simulink library "UXFD_Lib"  (R2016b)
settings: Solver=ode45  StartTime=0.0  StopTime=10.0  RelTol=1e-3  EnableMultiTasking=on
undefined symbols (not defined in the file): BreakpointData, BreakpointData1, BreakpointData2, BreakpointData_One_A, BreakpointData_Two_A, E2E_P01DataIDMode, E2E_P01ReceiverStatusType, EnumClass, iBit, initalValue, No_Runnable_Period, ObB_EidBsgStDerat_C, p_OVERRIDE_MASTER_SWITCH, SlDemoSign, SwitchOff_P, SwitchOn_P, Table, TableData_M, VCCTi33, VSysD_FidVehDerat1_C
libraries: simulink x28, CCMLib x11, UXFD_Lib x8, canmsglib x2, PTCC_Lib x1, hdlsllib x1
(part 1 of 7)
settings Model: Creator=yaqi.zheng  LastModifiedBy=jichang.liu
settings DataIOCC: LimitDataPoints=on
settings OptimizationCC: LifeSpan=inf
settings DebuggingCC: AllowSymbolicDim=off  SFUnexpectedBacktrackingDiag=warning  SFNoUnconditionalDefaultTransitionDiag=warning  SFExecutionAtInitializationDiag=none
settings GRTTargetCC: TargetLangStandard=C89/C90 (ANSI)  GeneratePreprocessorConditionals=Disable all
settings ConfigComp: CovMetricSettings=dw  CovHtmlReporting=on  CovSaveCumulativeToWorkspaceVar=on  CovSaveSingleToWorkspaceVar=on  CovExternalEMLEnable=off

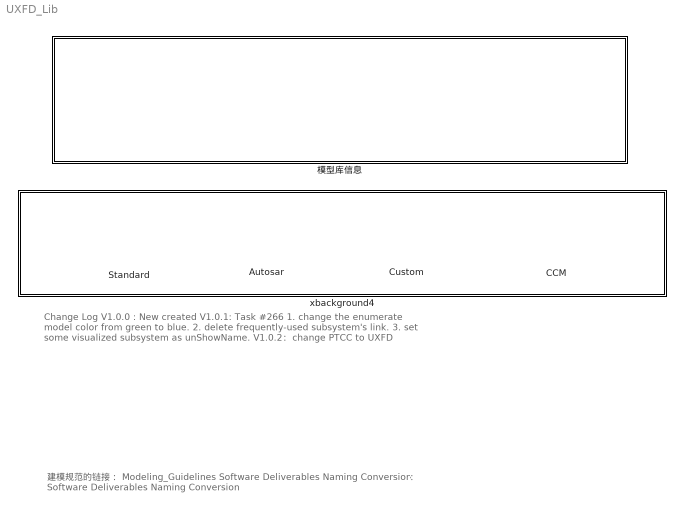
== system UXFD_Lib ==
  note: Change Log
      | V1.0.0 : New created
      |
      | V1.0.1: Task #266
      | 1. change the enumerate model color from green to blue.
      | 2. delete frequently-used subsystem's link.
      | 3. set some visualized subsystem as unShowName.
      | V1.0.2：
      | change PTCC to UXFD
  note: 建模规范的链接：
      | Modeling_Guidelines
      | Software Deliverables Naming Conversion：
      | Software Deliverables Naming Conversion
  Autosar : Subsystem
      mask Display: disp('Autosar')
  CCM : Subsystem
      mask Display: disp('CCM')
  Custom : Subsystem
      mask Display: disp('Custom')
  Standard : Subsystem
      mask Display: disp('Standard')
  xbackground4 : Subsystem
      mask Display: disp(' ')
  模型库信息 : Subsystem  mask(ModelHeader){prj=Geely, desc=UXFD 模型库, ver=1.0.2, date=2019.06.14, rev=0, author=UXFD, matlabver=MATLAB 2016a, simulinkver=MATLAB 2016a, stateflowver=0}
      mask prompts: prj "Project"; desc "Description"; ver "Version"; matlabver "MATLAB Ver"; simulinkver "Simulink Ver"; stateflowver "Stateflow Ver"
      mask init:
      | set_param(gcb, 'LinkStatus', 'none');
      mask Display:
      | plot([0 0 1 1 0],[0.03 1 1 0.03 0.03]) % 内层方框
      | plot([0.5 1],[0.85 0.85]) % 第一条横线
      | plot([0.5 1],[0.7 0.7]) % 第二条横线
      | plot([0.5 1],[0.55 0.55]) % 第三条线横线
      | plot([0.5 1],[0.4 0.4]) % 第四条线横线
      | plot([0 1],[0.25 0.25]) % 第五条横线
      | 
      | plot([0.5 0.5],[0.25 1]) % 第一条竖线
      | plot([0.60 0.60],[0.25 1])% 第二条竖线
      | plot([0.75 0.75],[0.25 1]) % 第三条竖线
      | plot([0.84 0.84],[0.25 1])% 第四条竖线
      | image(imread('geely.png','png'),[0.16 0.33 0.15 0.53]) % 图形位置
      | 
      | text(0.51,0.96,['\fontsize{8}\fontname{Times}\bfProject:'],'verticalAlignment','Top','horizontalAlignment','Left','texmode','on');
      | text(0.62,0.96,['\fontsize{8}\fontname{Times}\rm\fontsize{9}\fontsize{9}' prj],'verticalAlignment','Top','horizontalAlignment','Left','texmode','on');
      | 
      | text(0.51,0.81,['\fontsize{8}\fontname{Times}\bfVersion:' ],'verticalAlignment','Top','horizontalAlignment','Left','texmode','on');
      | text(0.62,0.81,['\fontsize{8}\fontname{Times}' ver],'verticalAlignment','Top','horizontalAlignment','Left','texmode','on');
      | 
      | text(0.51,0.67,['\fontsize{8}\fontname{Times}\bfDate:' ],'verticalAlignment','Top','horizontalAlignment','Left','texmode','on');
      | text(0.62,0.67,['\fontsize{8}\fontname{Times}\rm\fontsize{9}\fontsize{9}' date],'verticalAlignment','Top','horizontalAlignment','Left','texmode','on');
      | 
      | text(0.51,0.51,['\fontsize{8}\fontname{Times}\bfMATLAB Ver:' ],'verticalAlignment','Top','horizontalAlignment','Left','texmode','on');
      | text(0.62,0.51,['\fontsize{8}\fontname{Times}\rm\fontsize{9}\fontsize{9}' matlabver],'verticalAlignment','Top','horizontalAlignment','Left','texmode','on');
      | 
      | text(0.51,0.36,['\fontsize{8}\fontname{Times}\bfStateflow Ver:'],'verticalAlignment','Top','horizontalAlignment','Left','texmode','on');
      | text(0.62,0.36,['\fontsize{8}\fontname{Times}\rm\fontsize{9}\fontsize{9}' stateflowver],'verticalAlignment','Top','horizontalAlignment','Left','texmode','on');
      | %---------------------------------------------------------------------------------
      | text(0.76,0.96,['\fontsize{8}\fontname{Times}\bfAuthor:'],'verticalAlignment','Top','horizontalAlignment','Left','texmode','on');
      | text(0.86,0.96,['\fontsize{8}\fontname{Times}\rm\fontsize{9}\fontsize{9}' author],'verticalAlignment','Top','horizontalAlignment','Left','texmode','on');
      | 
      | text(0.76,0.81,['\fontsize{8}\fontname{Times}\bfRev:'],'verticalAlignment','Top','horizontalAlignment','Left','texmode','on');
      | text(0.86,0.81,['\fontsize{8}\fontname{Times}\rm\fontsize{9}\fontsize{9}' rev],'verticalAlignment','Top','horizontalAlignment','Left','texmode','on');
      | 
      | text(0.76,0.67,['\fontsize{8}\fontname{Times}\bfModel:'],'verticalAlignment','Top','horizontalAlignment','Left','texmode','on');
      | text(0.86,0.67,['\fontsize{8}\fontname{Times}\rm\fontsize{9}\fontsize{9}' desc],'verticalAlignment','Top','horizontalAlignment','Left','texmode','on');
      | 
      | text(0.76,0.51,['\fontsize{8}\fontname{Times}\bfSimulink Ver:'],'verticalAlignment','Top','horizontalAlignment','Left','texmode','on');
      | text(0.86,0.51,['\fontsize{8}\fontname{Times}\rm\fontsize{9}\fontsize{9}' simulinkver],'verticalAlignment','Top','horizontalAlignment','Left','texmode','on');
      | 
      | text(0.01,0.23,['\fontsize{8}\fontname{Times}\bfPROPRIETARY AND CONFIDENTIAL:\rm\fontsize{9}\newline\it\fontsize{10}\fontname{Arial}'                 'Geely Automobile Research Institute. All Right Reserved.'                 ],'verticalAlignment','Top','horizontalAlignment','Left','texmode','on');

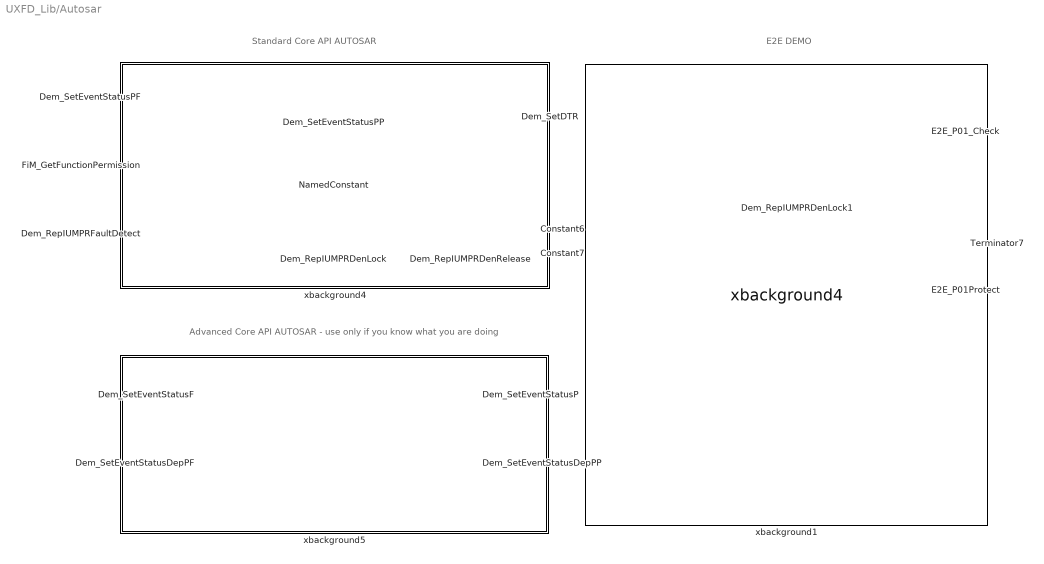
== system UXFD_Lib/Autosar ==
  note: Standard Core API AUTOSAR
  note: Advanced Core API AUTOSAR - use only if you know what you are doing
  note: E2E DEMO
  Constant6 : Constant  Value=72  OutDataTypeStr=Inherit: Inherit via back propagation
      settings: CopyFcn=set_param(gcbh,'ShowName','off');
  Constant7 : Constant  Value=220  OutDataTypeStr=Inherit: Inherit via back propagation
      settings: CopyFcn=set_param(gcbh,'ShowName','off');
  Dem_RepIUMPRDenLock : Subsystem  mask(Dem_RepIUMPRDenLock){}
      mask help: When enabled, this block will block the incrementation the denominator for Ratio Id Vc09XXXX.
      settings: AttributesFormatString=Dem_RepIUMPRDenLock
  Dem_RepIUMPRDenLock1 : PTCC_Lib/Autosar/Dem_RepIUMPRDenLock
      settings: AttributesFormatString=Dem_RepIUMPRDenLock
  Dem_RepIUMPRDenRelease : Subsystem  mask(Dem_RepIUMPRDenRelease){}
      mask help: When enabled, this block will release the incrementation the denominator for Ratio Id Vc09XXXX (i.e. if the conditions are fullfilled for incrementing the denominator for Ratio Id Vc09XXXX, it will be incremented).
      settings: AttributesFormatString=Dem_RepIUMPRDenRelease
  Dem_RepIUMPRFaultDetect : Subsystem  mask(Dem_RepIUMPRFaultDetect){}
      mask help: When enabled, report to the Core BSW, that Ratio Id Vc09XXXX has been able to detect a fault (increment Numerator for Ratio Id Vc09XXXX)
      settings: AttributesFormatString=Dem_RepIUMPRFaultDetect
  Dem_SetDTR : Subsystem  Description="API method to update mode $06 testdata.                                       Dem_SetDTR(UInt16 DTRId, sint32 TestVal, sint32 LowerLimit, sint32  UpperLimit, Ctrlval )"  mask(Vcc_SetDTR){lsb=1.0, offset=0}
      mask help:
      | Reports a DTR result with lower and upper limit.
      | The types of the TestValue and it limits should be Float32.
      | The test value and test limits are converted to Int32s using the
      | lsb and offset parameters in this block
      |
      | API is needed in OBD-relevant ECUs only
      settings: AttributesFormatString=Vcc_SetDTR
  Dem_SetEventStatusDepPF : Subsystem  TreatAsAtomicUnit=on  mask(Dem_SetEventStatusDepPre-Failed){}
      mask help:
      | Only to be used by dependability functions.
      | When enabled, events with status Pre-Failed is sent to the Diagnostic Core
      settings: AttributesFormatString=Dem_SetEventStatusDep\nPre-Failed
  Dem_SetEventStatusDepPP : Subsystem  TreatAsAtomicUnit=on  mask(Dem_SetEventStatusDepPre-Passed){}
      mask help:
      | Only to be used by dependability functions.
      | When enabled, events with status Pre-Passed is sent to the Diagnostic Core
      settings: AttributesFormatString=Dem_SetEventStatusDep\nPre-Passed
  Dem_SetEventStatusF : Subsystem  TreatAsAtomicUnit=on  mask(Dem_SetEventStatusFailed){}
      mask help: When enabled, events with status Failed is sent to the Diagnostic Core
      settings: AttributesFormatString=Dem_SetEventStatus\nFailed
  Dem_SetEventStatusP : Subsystem  mask(Dem_SetEventStatusPassed){}
      mask help: When enabled, events with status Passed is sent to the Diagnostic Core
      settings: AttributesFormatString=Dem_SetEventStatus\nPassed
  Dem_SetEventStatusPF : Subsystem  mask(Dem_SetEventStatusPre-Failed){}
      mask help: When enabled, events with status Pre-Failed is sent to the Diagnostic Core
      settings: AttributesFormatString=Dem_SetEventStatus\nPre-Failed
  Dem_SetEventStatusPP : Subsystem  mask(Dem_SetEventStatusPre-Passed){}
      mask help: When enabled, events with status Pre-Passed is sent to the Diagnostic Core
      settings: AttributesFormatString=Dem_SetEventStatus\nPre-Passed
  E2E_P01Protect : Subsystem
  E2E_P01_Check : Subsystem
  FiM_GetFunctionPermission : Subsystem  mask(FiM_GetFunctionPermission){}
      mask help:
      | When enabled, this block ask the core for permission to execute a monitor with the FID.
      | Note: If this is used for activating reconfigurations, Perm == 0 => Activate reconfiguration.
      settings: AttributesFormatString=FiM_GetFunctionPermission
  NamedConstant : Subsystem  mask(NamedConstant){const_name=VcEvName}
      mask prompts: const_name "Constant Name"
      mask help:
      | Enter a name for a preprocessor defined constant.
      | The following naming convention shall be used:
      | These prefixes shall be used for the following IDs (without underscores):
      | VcEv - Event IDs
      | VcFi - Function IDs (FiD)
      | VcRv - Ranking Value IDs
      | Vc06 - Mode $06 Test result IDs
      | Vc09 - IU(M)PR IDs (Mode $09)
      |
      | E.g.
      | VcEvBoostHigh - An event ID name for too high boost pressure
      | VcFiBoostPeak - A FiD for the Peak pressure boost monitor
      settings: AttributesFormatString=Named Constant
      mask Display: text(0.5, 0.5, get_param(gcb, 'const_name'), 'horizontalAlignment', 'center')
  Terminator7 : Terminator
  xbackground1 : UXFD_Lib/Autosar/xbackground4  SystemSampleTime=-1
  xbackground4 : Subsystem
      mask Display: disp(' ')
  xbackground5 : Subsystem
      mask Display: disp(' ')
  wires:
  E2E_P01Protect/1(E2E_P01Protect_ReturnType) -> Terminator7/1
  Constant6/1 -> E2E_P01Protect/1(DataLength)
  Constant7/1 -> E2E_P01Protect/2(DataID)

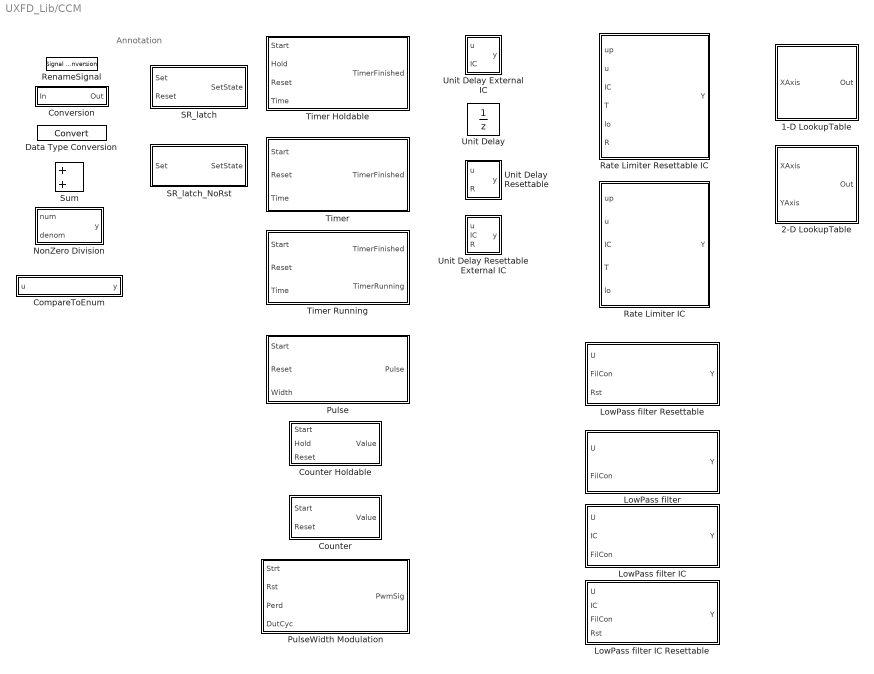
== system UXFD_Lib/CCM ==
  note: Annotation
  1-D LookupTable : Subsystem  mask(1D Lookup table NGCC v1.1){TableData=[4 7 6], TableDataDataType=Inherit: auto, BreakpointsXAxis=[1:3], BreakpointsXAxisDataType=Inherit: auto}
      mask help:
      | NGCC version of the Simulink standard 2-D lookup table.
      | "X-axis" is used as notation instead of "breakpoints 1".
      | Deviation from standard 2-D lookup table default settings:
      | - Extrapolation method: Clip, use last table value for inputs at or above last breakpoint.
      | - Saturate on integer overflow.
      | - Integer rounding mode: Floor
      | - Does NOT require all inputs to have the same data type
      |
      | Mx-VDev tested: Yes
      mask init:
      | blkNameMask = gcb;
      | 
      | % Redraw block at resize
      | set_param(blkNameMask,'MaskRunInitForIconRedraw','on')
      mask Display:
      | pos = get_param(gcb, 'Position');
      | width = pos(3) - pos(1);
      | height = pos(4) - pos(2);
      | doPlot = true;
      | blockHandle = gcb;
      | try
      |     tableDialogText = get_param(blockHandle,'TableData');
      |     try
      |         table = evalin('base',tableDialogText);
      |         tableValue = table.Value;
      |     catch
      |         tableValue = recursiveMaskParameterSearch(blockHandle,tableDialogText);
      |     end
      |     breakpointsXAxisDialogText = get_param(blockHandle,'BreakpointsXAxis');
      |     try
      |         breakpointsXAxisHandle = evalin('base',breakpointsXAxisDialogText);
      |         bp1 = breakpointsXAxisHandle.Value;
      |     catch
      |         bp1 = recursiveMaskParameterSearch(blockHandle,breakpointsXAxisDialogText);
      |     end
      | catch
      |     tableValue = str2num(get_param(blockHandle,'TableData'));
      |     bp1 = str2num(get_param(blockHandle,'BreakpointsXAxis'));
      |     doPlot = true;
      |     if (isempty(tableValue) || isempty(bp1))
      |         doPlot = false;
      |     end
      | end
      | if doPlot
      |     % Scale table and breakpoint data to fit block icon size
      |     if min(tableValue(:)) == max(tableValue(:))
      |         tableScaleTemp2 = ones(size(tableValue))*10;
      |     else
      |         tableScaleTemp1 = tableValue-min(tableValue(:));
      |         tableScaleTemp2 = (tableScaleTemp1/(max(tableScaleTemp1(:))-min(tableScaleTemp1(:))))*((height-5)-10);
      |     end
      |     tableScaled = tableScaleTemp2 + 5;
      | 
      |     if min(bp1(:)) == max(bp1(:))
      |         bp1ScaleTemp2 = bp1;
      |     else
      |         bp1ScaleTemp1 = bp1-min(bp1(:));
      |         bp1ScaleTemp2 = (bp1ScaleTemp1/(max(bp1ScaleTemp1(:))-min(bp1ScaleTemp1(:))))*((width-5)-12);
      |     end
      |     bp1Scaled = bp1ScaleTemp2 + 12;
      | 
      |     % plot data
      |     for i=1:length(tableValue(:,1))
      |         try
      |             plot(bp1Scaled,tableScaled(i,:))
      |         catch
      |             disp(num2str(tableScaled(i,:)))
      |         end
      |     end
      | 
      | else
      |     disp('Input data\nError')
      | end
      | % plot axis
      | plot([12 12],[5 height-10])
      | plot([12 width-5],[5 5])
      | 
      | port_label('input',1,'X')
      | text(width/2-20,height-7,'1-D T(x)')
  2-D LookupTable : Subsystem  mask(2D Lookup table NGCC v1.1){TableData=[4 5 6;16 19 20;10 18 23], TableDataDataType=Inherit: auto, BreakpointsXAxis=[1:3], BreakpointsXAxisDataType=Inherit: auto, BreakpointsYAxis=[1:3], BreakpointsYAxisDataType=Inherit: auto}
      mask help:
      | NGCC version of the Simulink standard 2-D lookup table.
      | "X- and Y-axis" is used as notation instead of "breakpoints 1" and "breakpoints 2".
      | Deviation from standard 2-D lookup table default settings:
      | - Extrapolation method: Clip, use last table value for inputs at or above last breakpoint.
      | - Saturate on integer overflow.
      | - Integer rounding mode: Floor
      | - Does NOT require all inputs to have the same data type
      |
      | Mx-VDev tested: Yes
      mask init:
      | blkNameMask = gcb;
      | 
      | % Redraw block at resize
      | set_param(blkNameMask,'MaskRunInitForIconRedraw','on')
      mask Display:
      | pos = get_param(gcb, 'Position');
      | width = pos(3) - pos(1);
      | height = pos(4) - pos(2);
      | doPlot = true;
      | blockHandle = gcb;
      | try
      |     tableDialogText = get_param(blockHandle,'TableData');
      |     try
      |         table = evalin('base',tableDialogText);
      |         tableValue = table.Value;
      |     catch
      |         tableValue = recursiveMaskParameterSearch(blockHandle,tableDialogText);
      |     end
      |     breakpointsYAxisDialogText = get_param(blockHandle,'BreakpointsYAxis');
      |     try
      |         breakpointsYAxisHandle = evalin('base',breakpointsYAxisDialogText);
      |         bp2 = breakpointsYAxisHandle.Value;
      |     catch
      |         bp2 = recursiveMaskParameterSearch(blockHandle,breakpointsYAxisDialogText);
      |     end
      |     breakpointsXAxisDialogText = get_param(blockHandle,'BreakpointsXAxis');
      |     try
      |         breakpointsXAxisHandle = evalin('base',breakpointsXAxisDialogText);
      |         bp1 = breakpointsXAxisHandle.Value;
      |     catch
      |         bp1 = recursiveMaskParameterSearch(blockHandle,breakpointsXAxisDialogText);
      |     end
      | catch
      |     tableValue = str2num(get_param(blockHandle,'TableData'));
      |     bp2 = str2num(get_param(blockHandle,'BreakpointsYAxis'));
      |     bp1 = str2num(get_param(blockHandle,'BreakpointsXAxis'));
      |     doPlot = true;
      |     if (isempty(tableValue) || isempty(bp1) || isempty(bp2))
      |         doPlot = false;
      |     end
      | end
      | if doPlot
      |     % Scale table and breakpoint data to fit block icon size
      |     if min(tableValue(:)) == max(tableValue(:))
      |         tableScaleTemp2 = ones(size(tableValue))*10;
      |     else
      |         tableScaleTemp1 = tableValue-min(tableValue(:));
      |         tableScaleTemp2 = (tableScaleTemp1/(max(tableScaleTemp1(:))-min(tableScaleTemp1(:))))*((height-5)-10);
      |     end
      |     tableScaled = tableScaleTemp2 + 5;
      | 
      |     if min(bp1(:)) == max(bp1(:))
      |         bp1ScaleTemp2 = bp1;
      |     else
      |         bp1ScaleTemp1 = bp1-min(bp1(:));
      |         bp1ScaleTemp2 = (bp1ScaleTemp1/(max(bp1ScaleTemp1(:))-min(bp1ScaleTemp1(:))))*((width-5)-12);
      |     end
      |     bp1Scaled = bp1ScaleTemp2 + 12;
      | 
      |     % plot data
      |     for i=1:length(tableValue(:,1))
      |         try
      |             plot(bp1Scaled,tableScaled(i,:))
      |         catch
      |             disp(num2str(tableScaled(i,:)))
      |         end
      |     end
      | 
      | else
      |     disp('Input data\nError')
      | end
      | % plot axis
      | plot([12 12],[5 height-10])
      | plot([12 width-5],[5 5])
      | 
      | port_label('input',1,'X')
      | port_label('input',2,'Y')
      | text(width/2-20,height-7,'2-D T(x,y)')
  CompareToEnum : Subsystem  mask(Compare to Enum NGCC v1.0){relop===, const=EnumClass.Value, OutDataTypeStr=boolean, ZeroCross=on}
      mask prompts: relop "Simulink:masks:Operator_MP"; const "Simulink:masks:ConstantValue_MP"; OutDataTypeStr "Simulink:masks:OutputDataType_MP"; ZeroCross "Simulink:masks:EnableZerocrossingDetection_MP"
      mask help:
      | Compare to an Enum. Enum class is hidden from the mask i.e. displays only the value if the Enum is defined.
      |
      | Mx-VDev tested: Yes
      mask init:
      | blkName = gcb;
      | 
      | if strcmp(get_param(gcbh,'OutDataTypeStr'),'boolean')
      | 	setValue = 'boolean';
      | else
      | 	setValue = 'fixdt(0, 8)';
      | end
      | 
      | set_param([blkName,'/Compare'],'relop',relop, ...
      | 	'OutDataTypeStr', setValue, 'ZeroCross', ZeroCross);
      | 
      | str = [relop,' C']; %default
      | 
      | const_str = get_param(blkName, 'const');
      | 
      | if isempty(strfind(const_str, ' ')) && isempty(strfind(const_str, ','))
      |     % scalar or single expression
      |     if isempty(str2num(const_str))
      |         %expression
      |         str = [relop, ' ', const_str];
      |     elseif length(const) == 1
      |         if ismethod(const,'addClassNameToEnumNames') % Enum
      |             str = [relop,' ',char(const)];
      |         else
      |             str = [relop,' ',num2str(double(const))];
      |         end
      |     end
      | end
      mask TypeOptions relop: == | ~= | < | <= | >= | >
      mask TypeOptions OutDataTypeStr: uint8 | boolean
      mask Callback ZeroCross: sl('zeroCrossEnable', gcbh);
      mask Display: disp(str)
  Conversion : Subsystem  mask(Data Type Conversion NGCC v1.1){outputDataType=Inherit: Inherit via back propagation}
      mask prompts: outputDataType "Convert data type to:"
      mask help:
      | CCM version of the standard Simulink block.
      | This version displays the output data type name on the block icon, regardless of data type.
      |
      | Mx-VDev tested: Yes
      mask Display:
      | if strcmp(char(get_param(gcb,'MaskValues')),'Inherit: Inherit via back propagation')
      |     disp('Conversion')
      | else
      |     disp(char(get_param(gcb,'MaskValues')))
      | end
  Counter : Subsystem  mask(Counter NGCC v1.0){}
      mask help:
      | If Start (1) is true, the counter is started.
      | Counter will be reset to 0 and stopped if Reset (2) is true.
      | This block is reset dominant.
      | Value (output) specifies the counter value, data type VCCUInt32.
      |
      | Mx-VDev tested: Yes
      mask Display:
      | try
      |     image(imread([CCMConfig.GetRootDir '\Shared\SimulinkLibrary\Images\counter.bmp']))
      | catch
      |     fprintf('Counter\nHoldable')
      | end
      | port_label('output',1,'Value')
      | port_label('input',1,'Start')
      | port_label('input',2,'Reset')
  Counter Holdable : Subsystem  mask(Counter Holdable NGCC v1.0){}
      mask help:
      | If Start (1) is true, the counter is started.
      | Counter will continue counting until Hold (2) is true, then the counter value will be held.
      | Counter will be reset to 0 if Reset (3) is true.
      | Value (output) specifies the counter value, data type VCCUInt32.
      |
      | Mx-VDev tested: Yes
      mask Display:
      | try
      |     image(imread([CCMConfig.GetRootDir '\Shared\SimulinkLibrary\Images\counter.bmp']))
      | catch
      |     fprintf('Counter\nHoldable')
      | end
      | port_label('output',1,'Value')
      | port_label('input',1,'Start')
      | port_label('input',2,'Hold')
      | port_label('input',3,'Reset')
  Data Type Conversion : DataTypeConversion  SaturateOnIntegerOverflow=on
      settings: AttributesFormatString=%<OutDataTypeStr>
  LowPass filter : Subsystem  mask(Low-pass filter NGCC v1.0){InputOutputDataType=single, FilterConstantDataType=VCCTi33, RunnablePeriod=No_Runnable_Period}
      mask prompts: InputOutputDataType "Input/Output Data Type"; FilterConstantDataType "Filter Time Constant Data Type:"; RunnablePeriod "SWC Sampling Time Parameter:"
      mask help:
      | Typical NGCC low-pass filter with filter length 1.
      | U is the input signal that is to be filtered.
      | FilCon is the filter time constant.
      | Y is the filtered output.
      |
      | Mx-VDev tested: Yes
      mask init:
      | blkNameMask = gcb;
      | IODataType = get_param(blkNameMask,'InputOutputDataType');
      | if strcmp(IODataType,'single')
      |     dataTypeSlope = 2^(-12);
      | else
      |     try
      |     dataTypeSlope = evalin('base',[IODataType '.Slope']); %Fixed point
      |     catch
      |         dataTypeSlope = 1; %Integer
      |     end
      | end
      | %Set sampletime
      | blkName = gcb;
      | modelName = char(regexp(blkName,'(\w*)_(?:Runnable|lib)','tokens','once'));
      | if isempty(modelName)
      |     modelName = 'No';
      | end
      | timeParameter = [modelName '_Runnable_Period'];
      | set_param(blkName, 'RunnablePeriod',timeParameter);
      mask Display: disp(['Y = U[n]*k + Y[n-1]*(1-k)' char(uint16(10)) 'n: sample' char(uint16(10)) 'k: filter constant' char(uint16(10)) 'Init value = U[0]']);
  LowPass filter Resettable : Subsystem  mask(Low-pass filter Resettable NGCC v1.0){InputOutputDataType=single, FilterConstantDataType=VCCTi33, RunnablePeriod=No_Runnable_Period}
      mask prompts: InputOutputDataType "Input/Output Data Type"; FilterConstantDataType "Filter Time Constant Data Type:"; RunnablePeriod "SWC Sampling Time Parameter:"
      mask help:
      | Typical NGCC low-pass filter with filter length 1.
      | U is the input signal that is to be filtered.
      | FilCon is the filter time constant.
      | Rst is the filter reset condition (boolean).
      | Y is the filtered output.
      |
      | Mx-VDev tested: Yes
      mask init:
      | %Set sample time
      | blkName = gcb;
      | modelName = char(regexp(blkName,'(\w*)_(?:Runnable|lib)','tokens','once'));
      | if isempty(modelName)
      |     modelName = 'No';
      | end
      | timeParameter = [modelName '_Runnable_Period'];
      | set_param(blkName, 'RunnablePeriod',timeParameter);
      mask Display: disp(['Y = U[n]*k + Y[n-1]*(1-k)' char(uint16(10)) 'n: sample' char(uint16(10)) 'k: filter constant' char(uint16(10)) 'Init value = U[0]']);
  LowPass filter IC : Subsystem  mask(Low-pass filter IC NGCC v1.0){InputOutputDataType=single, FilterConstantDataType=VCCTi33, RunnablePeriod=No_Runnable_Period}
      mask prompts: InputOutputDataType "Input/Output Data Type"; FilterConstantDataType "Filter Time Constant Data Type:"; RunnablePeriod "SWC Sampling Time Parameter:"
      mask help:
      | Typical NGCC low-pass filter with filter length 1.
      | U is the input signal that is to be filtered.
      | IC is the initial condition value.
      | FilCon is the filter time constant.
      | Y is the filtered output.
      |
      | Mx-VDev tested: No
      mask init:
      | blkNameMask = gcb;
      | IODataType = get_param(blkNameMask,'InputOutputDataType');
      | if strcmp(IODataType,'single')
      |     dataTypeSlope = 2^(-12);
      | else
      |     try
      |     dataTypeSlope = evalin('base',[IODataType '.Slope']); %Fixed point
      |     catch
      |         dataTypeSlope = 1; %Integer
      |     end
      | end
      | 
      | %Set sample time
      | blkName = gcb;
      | modelName = char(regexp(blkName,'(\w*)_(?:Runnable|lib)','tokens','once'));
      | if isempty(modelName)
      |     modelName = 'No';
      | end
      | timeParameter = [modelName '_Runnable_Period'];
      | set_param(blkName, 'RunnablePeriod',timeParameter);
      mask Display: disp(['Y = U[n]*k + Y[n-1]*(1-k)' char(uint16(10)) 'n: sample' char(uint16(10)) 'k: filter constant' char(uint16(10)) 'Init value = IC']);
  LowPass filter IC Resettable : Subsystem  mask(Low-pass filter IC Resettable NGCC v1.0){InputOutputDataType=single, FilterConstantDataType=VCCTi33, RunnablePeriod=No_Runnable_Period}
      mask prompts: InputOutputDataType "Input/Output Data Type"; FilterConstantDataType "Filter Time Constant Data Type:"; RunnablePeriod "SWC Sampling Time Parameter:"
      mask help:
      | Typical NGCC low-pass filter with filter length 1.
      | IC is the initial condition (value).
      | U is the input signal that is to be filtered.
      | FilCon is the filter time constant.
      | Rst is the filter reset condition (boolean).
      | Y is the filtered output.
      |
      | Mx-VDev tested: No
      mask init: same as UXFD_Lib/CCM/LowPass filter Resettable
      mask Display: disp(['Y = U[n]*k + Y[n-1]*(1-k)' char(uint16(10)) 'n: sample' char(uint16(10)) 'k: filter constant' char(uint16(10)) 'Init value = IC']);
  NonZero Division : Subsystem  mask(Non Zero Division NGCC v1.3){dataTypeNum=single, dataTypeDen=single, dataTypeOut=single}
      mask prompts: dataTypeNum "Data type of numerator"; dataTypeDen "Data type of denominator"; dataTypeOut "Data type of output"
      mask help:
      | Performs a division that is protected against division by zero.
      | First input is numerator, second input is denominator.
      | User must enter the data types of the two input signals as well as the output signal.
      |
      | Mx-VDev tested: Yes
      mask init:
      | blkNameMask = gcb;
      | DenominatorDataType = get_param(blkNameMask,'dataTypeDen');
      | if strcmp(DenominatorDataType,'single')
      |     dataTypeSlope = 2^(-100);
      | else
      |     try
      |         dataTypeSlope = evalin('base',[DenominatorDataType '.Slope']); %Fixed point
      |     catch
      |         dataTypeSlope = 1; %Integer
      |     end
      | end
      mask Display:
      | port_label('output',1,'y')
      | port_label('input',1,'x')
      | port_label('input',2,'÷')
      | fprintf('Non-Zero\nDivision')
  Pulse : Subsystem  mask(Pulse NGCC v1.0){timeDataType=VCCTi33, RunnablePeriod=No_Runnable_Period}
      mask prompts: timeDataType "Pulse width data type (s):"; RunnablePeriod "SWC Sampling Time Parameter:"
      mask help:
      | If Start (1) is true, the Pulse (output) is started.
      | If Start is set during [Pulse == true], the timer is reset and the Pulse is kept true.
      | Pulse will be reset to 0 if Reset (2) is true.
      | Width (3) defines the pulse width in seconds.
      | If Width is set to zero, Pulse will be set to false.
      | Reset is always master over Start.
      |
      | Mx-VDev tested: Yes
      mask init: same as UXFD_Lib/CCM/LowPass filter Resettable
      mask Display:
      | x=[0.2 0.35 0.35 0.65 0.65 0.8];
      | y=[0.2 0.2 0.7 0.7 0.2 0.2];
      | plot(x,y)
  PulseWidth Modulation : Subsystem  mask(PulseWidth Modulation NGCC v1.0){timeDataType=VCCTi33, RunnablePeriod=No_Runnable_Period}
      mask prompts: timeDataType "Period time input data type:"; RunnablePeriod "SWC Sampling Time Parameter:"
      mask help:
      | If Start(1) is true the pulse generator is started.
      | It will continue to run until Reset(2) is true. It will start again when Reset is set to false.
      | Data type of Period time(3) and the SWC Sampling Time has to be specified in the mask.
      | Data type of Duty Cycle(4) is VCCPerc30 and determines the ratio of the period time when the signal is true.
      | The period starts with the duty cycle, i.e. the signal is first true after reset or start.
      | Default value, when pulse generator is not started or when it is held with the reset function, is true.
      |
      | Mx-VDev tested: Yes
      mask init: same as UXFD_Lib/CCM/LowPass filter Resettable
      mask Display:
      | x=[0.1 1 1 2.1 2.1 3 3 4.1 4.1 5 5 6.1 6.1 7 7 8.1] * 10 + 30;
      | y=[1 1 0 0 1 1 0 0 1 1 0 0 1 1 0 0] * 15 + 30;
      | plot(x,y)
  Rate Limiter IC : Subsystem  mask(Rate Limiter Dynamic IC NGCC v1.0){InputOutputDataType=single}
      mask prompts: InputOutputDataType "Data type inputs/output:"
      mask help:
      | Limit rising and falling rates of the input signal.
      | up: upper rate limit
      | u: input signal to be rate limited
      | IC: initial condition
      | T: SWC runnable period
      | lo: lower rate limit (input should be negative)
      |
      | The rates 'up' and 'lo' should be per second (*/s), since the block converts seconds to sample before calculations.
      |
      | Mx-VDev tested: Yes
      mask Display: plot([0.15 0.95],[.5 .5],[.5 .5],[0.05 0.95],0.05+0.9*[.2 .8],0.05+0.9*[0 1]);
  Rate Limiter Resettable IC : Subsystem  mask(Rate Limiter Dynamic Resettable IC NGCC v1.0){InputOutputDataType=single}
      mask prompts: InputOutputDataType "Data type inputs/output:"
      mask help:
      | Limit rising and falling rates of the input signal.
      | up: upper rate limit
      | u: input signal to be rate limited
      | IC: initial condition
      | T: SWC runnable period
      | lo: lower rate limit
      | R: reset flag, resets to the initial condition
      |
      | The rates 'up' and 'lo' should be per second (*/s), since the block converts seconds to sample before calculations.
      |
      | Mx-VDev tested: Yes
      mask Display: plot([0.15 0.95],[.5 .5],[.5 .5],[0.05 0.95],0.05+0.9*[.2 .8],0.05+0.9*[0 1]);
  RenameSignal : SignalConversion  OverrideOpt=on  mask(Rename signal NGCC v1.1){}
      mask help:
      | Typically used when bus signals are relayed.
      |
      | Mx-VDev tested: Yes
      mask Display: fprintf('Rename')
  SR_latch : Subsystem  mask(SR-latch NGCC v1.0){}
      mask help:
      | Set/reset-latch with default value 0 (false).
      | S   R   Q
      | ----------
      | 0   0   Q[n-1]
      | 0   1   0
      | 1   0   1
      | 1   1   0
      |
      | where Q[n-1] is the previous output value.
      |
      | Mx-VDev tested: Yes
  SR_latch_NoRst : Subsystem  mask(SR-latch-no-reset NGCC v1.0){}
      mask help:
      | Set-latch with default value 0 (false).
      | S   Q
      | ----------
      | 0   Q[n-1]
      | 1   1
      |
      | where Q[n-1] is the previous output value.
      |
      | Mx-VDev tested: Yes
  Sum : Sum  SaturateOnIntegerOverflow=on  InputSameDT=on
  Timer : Subsystem  mask(Timer NGCC v1.0){timeDataType=VCCTi33, RunnablePeriod=No_Runnable_Period}
      mask prompts: timeDataType "Time data type:"; RunnablePeriod "SWC Sampling Time Parameter:"
      mask help:
      | If Start (1) is true, the timer is started.
      | The timer works as a "set/reset"-functionality, i.e. start does not have to be "true" continuously to keep the timer running.
      | Timer will be reset to 0 if Reset (2) is true.
      | TimerFinished (output) specifies if the timer is finished (boolean).
      | If Time (3) is set to zero, this block will function as a set-reset latch.
      | Reset is always master over Start.
      |
      | Mx-VDev tested: Yes
      mask init: same as UXFD_Lib/CCM/LowPass filter Resettable
      mask Display:
      | try
      |     image(imread([CCMConfig.GetRootDir '\Shared\SimulinkLibrary\Images\timer.bmp']))
      | catch
      |     fprintf('Timer\nHoldable')
      | end
      | port_label('output',1,'TmrFinshd')
      | port_label('input',1,'Start')
      | port_label('input',2,'Reset')
      | port_label('input',3,'Time')
  Timer Holdable : Subsystem  mask(Timer Holdable NGCC v1.1){timeDataType=VCCTi33, RunnablePeriod=No_Runnable_Period}
      mask prompts: timeDataType "Time data type:"; RunnablePeriod "SWC Sampling Time Parameter:"
      mask help:
      | If Start (1) is true, the timer is started.
      | Timer will continue running until Hold (2) is true, then the timer value will be held.
      | If Hold becomes false, the timer will continue when conditions to start is fulfilled.
      | The Start and Hold serve as a "set/reset"-functionality, i.e. start does not have to be "true" continuously to keep the timer running.
      | Timer will be reset to 0 if Reset (3) is true.
      | TimerFinished (output) specifies if the timer is finished (boolean).
      | If Time is set to zero, this block will function as a set-reset latch.
      | Hold and Reset are always master over Start.
      |
      | Mx-VDev tested: Yes
      mask init: same as UXFD_Lib/CCM/LowPass filter Resettable
      mask Display:
      | try
      |     image(imread([CCMConfig.GetRootDir '\Shared\SimulinkLibrary\Images\timer.bmp']))
      | catch
      |     fprintf('Timer\nHoldable')
      | end
      | port_label('output',1,'TmrFinshd')
      | port_label('input',1,'Start')
      | port_label('input',2,'Hold')
      | port_label('input',3,'Reset')
      | port_label('input',4,'Time')
  Timer Running : Subsystem  mask(Timer Running NGCC v1.0){timeDataType=VCCTi33, RunnablePeriod=No_Runnable_Period}
      mask prompts: timeDataType "Time data type:"; RunnablePeriod "SWC Sampling Time Parameter:"
      mask help:
      | If Start (1) is true, the timer is started.
      | The timer works as a "set/reset"-functionality, i.e. start does not have to be "true" continuously to keep the timer running.
      | Timer will be reset to 0 if Reset (2) is true.
      | TimerFinished (output) specifies if the timer is finished (boolean).
      | If Time (3) is set to zero, this block will function as a set-reset latch.
      | Reset is always master over Start.
      |
      | TmrRunng (output 2) will be set when timer is activated.
      |
      | Mx-VDev tested: Yes
      mask init: same as UXFD_Lib/CCM/LowPass filter Resettable
      mask Display:
      | try
      |     image(imread([CCMConfig.GetRootDir '\Shared\SimulinkLibrary\Images\timer.bmp']))
      | catch
      |     fprintf('Timer\nHoldable')
      | end
      | port_label('output',1,'TmrFinshd')
      | port_label('output',2,'TmrRunng')
      | port_label('input',1,'Start')
      | port_label('input',2,'Reset')
      | port_label('input',3,'Time')
  Unit Delay : UnitDelay  InitialCondition=initalValue  SampleTime=-1
      settings: AttributesFormatString=X0=%<X0>
  Unit Delay External IC : Subsystem  mask(Unit Delay External Initial Condition NGCC v1.0){dataType=single}
      mask prompts: dataType "Data type:"
      mask help:
      | NGCC version of the Simulink built-in block with data type control and boolean datatype usage for internal switch condition.
      | -----------------------------------------------------
      | Normally, the output is the signal u delayed by one sample period.
      | The initial condition is given by the signal IC.
      |
      | Mx-VDev tested: Yes
      mask Display: dpoly(1,[1 0],'z')
  Unit Delay Resettable : Subsystem  mask(Unit Delay Resettable NGCC v1.0){initialCondition=0, dataType=single}
      mask prompts: initialCondition "Initial condition:"; dataType "Data type:"
      mask help:
      | NGCC version of the Simulink built-in block with data type control and boolean datatype usage for internal switch condition.
      | -----------------------------------------------------
      | Normally, the output is the signal u delayed by one sample period.
      | When the reset signal R is true, the state and the output are always set equal to the initial condition parameter.  This reset action is vectorized and supports scalar expansion.
      |
      | Mx-VDev tested: Yes
      settings: AttributesFormatString=X0=%<initialCondition>
      mask Display: dpoly(1,[1 0],'z')
  Unit Delay Resettable External IC : Subsystem  mask(Unit Delay Resettable External Initial Condition NGCC v1.0){dataType=single}
      mask prompts: dataType "Data type:"
      mask help:
      | NGCC version of the Simulink built-in block with data type control and boolean datatype usage for internal switch condition.
      | -----------------------------------------------------
      | Normally, the output is the signal u delayed by one sample period.
      | When the reset signal R is true, the state and the output are always set equal to the initial condition signal IC.  This reset action is vectorized and supports scalar expansion.
      |
      | Mx-VDev tested: Yes
      mask Display: dpoly(1,[1 0],'z')

== system UXFD_Lib/Custom ==
  CAN : Subsystem
      mask Display: disp('CAN')
  Diagnose : Subsystem
      mask Display: disp('Diagnose')
  PIN : Subsystem
      mask Display: disp('PIN')
  xbackground4 : UXFD_Lib/xbackground4  SystemSampleTime=-1

== system UXFD_Lib/Standard ==
  Bit Operation : Subsystem
      settings: CopyFcn=set_param(gcbh,'ShowName','off');
      mask Display: disp('Bit Operation')
  Calibration : Subsystem
      settings: CopyFcn=set_param(gcbh,'ShowName','off');
      mask Display: disp('Calibration')
  Discrete dynamics : Subsystem
      settings: CopyFcn=set_param(gcbh,'ShowName','off');
      mask Display: disp('Discrete dynamics')
  Math : Subsystem
      mask Display: disp('Math')
  Relation&Logic : Subsystem
      mask Display: disp('Relation & Logic')
  Signals and systems : Subsystem
      mask Display: disp('Signals and systems')
  xbackground4 : UXFD_Lib/xbackground4  SystemSampleTime=-1

== system UXFD_Lib/xbackground4 ==

== system UXFD_Lib/模型库信息 ==

== system UXFD_Lib/Autosar/Dem_RepIUMPRDenLock ==
  Vc09 : Inport
  EntryCond : EnablePort
  Dem_RepIUMPRDenLock : S-Function  FunctionName=Dem_RepIUMPRDenLock_flp  Parameters=dt  SFunctionDeploymentMode=off  EnableBusSupport=off  mask(TL_CustomCode){data={'#state',0,'#param',0,'#work',0,'codefile','Dem_RepIUMPRDenLock.c','prodcode',0,'logdata',{'plotchannels',[]},'output',{'name','$S_ok','varname','ok','type','Bool'},'input',{'name','$S_RatioId','varname','RatioId','type','UInt16'},'date',735300.29244876152}, dt=-1}
      mask help:
      | TargetLink Custom Code block:
      | Allows to insert custom code into a TargetLink application.
      settings: AttributesFormatString=Dem_RepIUMPRDenLock  DeleteFcn=if exist('delete_tlblock','file')==2,delete_tlblock(gcbh);end  NameChangeFcn=if exist('rename_tlblock','file')==2,rename_tlblock(gcbh);end  OpenFcn=if exist('tl_open_blockdlg','file')==2,tl_open_blockdlg(gcbh);else,open_system(gcbh,'mask');end
      mask Help: eval(['tl_online_help(''Topic'',''',get_param(gcbh,'MaskType'),''')'])
      mask Display:
      | plot([-0.05, 1.05, NaN, -0.05, 1.05],[.01, .01, NaN, .99, .99])
      | ; disp('Dem_RepIUMPRDenLock.c');port_label('input',1,'RatioId');port_label('output',1,'ok');
  Terminator3 : Terminator
  wires:
  Vc09/1 -> Dem_RepIUMPRDenLock/1
  Dem_RepIUMPRDenLock/1 -> Terminator3/1

== system UXFD_Lib/Autosar/Dem_RepIUMPRDenRelease ==
  Vc09 : Inport
  EntryCond : EnablePort
  Dem_RepIUMPRDenRelease : S-Function  FunctionName=Dem_RepIUMPRDenRelease_flp  Parameters=dt  SFunctionDeploymentMode=off  EnableBusSupport=off  mask(TL_CustomCode){data={'#state',0,'#param',0,'#work',0,'codefile','Dem_RepIUMPRDenRelease.c','prodcode',0,'logdata',{'plotchannels',[]},'output',{'name','$S_ok','varname','ok','type','Bool'},'input',{'name','$S_RatioId','varname','RatioId','type','UInt16'},'date',735300.29243282403}, dt=-1}
      mask help:
      | TargetLink Custom Code block:
      | Allows to insert custom code into a TargetLink application.
      settings: AttributesFormatString=Dem_RepIUMPRDenRelease  DeleteFcn=if exist('delete_tlblock','file')==2,delete_tlblock(gcbh);end  NameChangeFcn=if exist('rename_tlblock','file')==2,rename_tlblock(gcbh);end  OpenFcn=if exist('tl_open_blockdlg','file')==2,tl_open_blockdlg(gcbh);else,open_system(gcbh,'mask');end
      mask Help: eval(['tl_online_help(''Topic'',''',get_param(gcbh,'MaskType'),''')'])
      mask Display:
      | plot([-0.05, 1.05, NaN, -0.05, 1.05],[.01, .01, NaN, .99, .99])
      | ; disp('Dem_RepIUMPRDenRelease.c');port_label('input',1,'RatioId');port_label('output',1,'ok');
  Terminator3 : Terminator
  wires:
  Dem_RepIUMPRDenRelease/1 -> Terminator3/1
  Vc09/1 -> Dem_RepIUMPRDenRelease/1

== system UXFD_Lib/Autosar/Dem_RepIUMPRFaultDetect ==
  Vc09 : Inport
  EntryCond : EnablePort
  Dem_RepIUMPRFaultDetect : S-Function  FunctionName=Dem_RepIUMPRFaultDetect_flp  Parameters=dt  SFunctionDeploymentMode=off  EnableBusSupport=off  mask(TL_CustomCode){data={'#state',0,'#param',0,'#work',0,'codefile','Dem_RepIUMPRFaultDetect.c','prodcode',0,'logdata',{'plotchannels',[]},'output',{'name','$S_ok','varname','ok','type','Bool'},'input',{'name','$S_RatioId','varname','RatioId','type','UInt16'},'date',735300.29241528932}, dt=-1}
      mask help:
      | TargetLink Custom Code block:
      | Allows to insert custom code into a TargetLink application.
      settings: AttributesFormatString=Dem_RepIUMPRFaultDetect  DeleteFcn=if exist('delete_tlblock','file')==2,delete_tlblock(gcbh);end  NameChangeFcn=if exist('rename_tlblock','file')==2,rename_tlblock(gcbh);end  OpenFcn=if exist('tl_open_blockdlg','file')==2,tl_open_blockdlg(gcbh);else,open_system(gcbh,'mask');end
      mask Help: eval(['tl_online_help(''Topic'',''',get_param(gcbh,'MaskType'),''')'])
      mask Display:
      | plot([-0.05, 1.05, NaN, -0.05, 1.05],[.01, .01, NaN, .99, .99])
      | ; disp('Dem_RepIUMPRFaultDetect.c');port_label('input',1,'RatioId');port_label('output',1,'ok');
  Terminator3 : Terminator
  wires:
  Dem_RepIUMPRFaultDetect/1 -> Terminator3/1
  Vc09/1 -> Dem_RepIUMPRFaultDetect/1

== system UXFD_Lib/Autosar/Dem_SetDTR ==
  Vc06 : Inport
  TestVal : Inport  Port=2
  UpperLim : Inport  Port=3
  LowerLim : Inport  Port=4
  EntryCond : EnablePort
  Constant : Constant  Value=lsb  mask(TL_Constant){data={'output',{'type','Float32'},'date',736225.32098471059}}
      settings: CopyFcn=if exist('tl_reset_reviewflag','file')==2,tl_reset_reviewflag(gcbh);end  DeleteFcn=if exist('delete_tlblock','file')==2,delete_tlblock(gcbh);end  NameChangeFcn=if exist('rename_tlblock','file')==2,rename_tlblock(gcbh);end  OpenFcn=if exist('tl_open_blockdlg','file')==2,tl_open_blockdlg(gcbh);else,open_system(gcbh,'parameter');end
      mask Help: eval(['if exist(''tl_online_help'',''file'') == 2, tl_online_help(''Topic'',''TL_Constant''),else, web([''jar:file:///'',matlabroot,''/help/toolbox/simulink/help.jar!/slref/' lower(get_param(gcbh,'Blocktype')) '.html''], ''-helpbrowser''),end'])
      mask Display: plot([-0.05, 1.05, NaN, -0.05, 1.05],[.01, .01, NaN, .99, .99])
  Constant1 : Constant  Value=offset  mask(TL_Constant){data={'output',{'type','Float32'},'date',736225.32119465282}}
      settings: CopyFcn=if exist('tl_reset_reviewflag','file')==2,tl_reset_reviewflag(gcbh);end  DeleteFcn=if exist('delete_tlblock','file')==2,delete_tlblock(gcbh);end  NameChangeFcn=if exist('rename_tlblock','file')==2,rename_tlblock(gcbh);end  OpenFcn=if exist('tl_open_blockdlg','file')==2,tl_open_blockdlg(gcbh);else,open_system(gcbh,'parameter');end
      mask Help: eval(['if exist(''tl_online_help'',''file'') == 2, tl_online_help(''Topic'',''TL_Constant''),else, web([''jar:file:///'',matlabroot,''/help/toolbox/simulink/help.jar!/slref/' lower(get_param(gcbh,'Blocktype')) '.html''], ''-helpbrowser''),end'])
      mask Display: plot([-0.05, 1.05, NaN, -0.05, 1.05],[.01, .01, NaN, .99, .99])
  Terminator4 : Terminator
  Vcc_SetDTR : S-Function  Description=|  FunctionName=Vcc_SetDTR_flp  Parameters=dt  SFunctionDeploymentMode=off  EnableBusSupport=off  mask(TL_CustomCode){data={'#state',0,'#param',0,'#work',0,'#input',6,'codefile','Vcc_SetDTR.c','prodcode',0,'output',{'name','$S_ok','varname','ok','type','UInt8'},'input#1',{'name','$S_TRID','varname','TRID','type','UInt16'},'input#2',{'name','$S_TestVal','varname','TestVal','type','Float32'},'input#3',{'name','$S_TestMaxLimit','varname','UpperLimit','type','Float32'},'input#4',{'name','$S_TestMinLimit','varname','LowerLimit','type','Float32'},'input#5',{'name','$S_lsb','varname','lsb','type','Float32'},'input#6',{'name','$S_offset','varname','offset','type','Float32'},'date',736225.31771384261}, dt=-1}
      | Reports a DTR result with lower and upper limit. The internal
      | eventstatus serves as master whether the DTR values are      
      | forwarded or ignored, also taking the DTRUpdateKind into     
      | account. The EventId that is related to the DTR is assigned  
      | per configuration (and derived from ServiceNeeds). Processing
      | takes enable/storage conditions into account. API            
      | is needed in OBD-relevant ECUs only
      mask help:
      | TargetLink Custom Code block:
      | Allows to insert custom code into a TargetLink application.
      settings: AttributesFormatString=Vcc_SetDTR  DeleteFcn=if exist('delete_tlblock','file')==2,delete_tlblock(gcbh);end  NameChangeFcn=if exist('rename_tlblock','file')==2,rename_tlblock(gcbh);end  OpenFcn=if exist('tl_open_blockdlg','file')==2,tl_open_blockdlg(gcbh);else,open_system(gcbh,'mask');end
      mask Help: eval(['tl_online_help(''Topic'',''',get_param(gcbh,'MaskType'),''')'])
      mask Display:
      | plot([-0.05, 1.05, NaN, -0.05, 1.05],[.01, .01, NaN, .99, .99])
      | ; disp('Vcc_SetDTR.c');port_label('input',1,'TRID');port_label('input',2,'TestVal');port_label('input',3,'UpperLimit');port_label('input',4,'LowerLimit');port_label('input',5,'lsb');port_label('input',6,'offset');port_label('output',1,'ok');
  wires:
  Constant1/1 -> Vcc_SetDTR/6
  Constant/1 -> Vcc_SetDTR/5
  Vcc_SetDTR/1 -> Terminator4/1
  LowerLim/1 -> Vcc_SetDTR/4
  UpperLim/1 -> Vcc_SetDTR/3
  TestVal/1 -> Vcc_SetDTR/2
  Vc06/1 -> Vcc_SetDTR/1

== system UXFD_Lib/Autosar/Dem_SetEventStatusDepPF ==
  VcEv : Inport
  EntryCond : EnablePort
  Dem_SetEventStatus : S-Function  FunctionName=Dem_SetEventStatusDep_flp  Parameters=dt  SFunctionDeploymentMode=off  EnableBusSupport=off  mask(TL_CustomCode){data={'#state',0,'#param',0,'#work',0,'#input',2,'codefile','Dem_SetEventStatusDep.c','prodcode',0,'logdata',{'plotchannels',[]},'output',{'name','$S_ok','varname','ok','type','Bool'},'input#1',{'name','$S_EventId','varname','EventId','type','UInt16'},'input#2',{'name','$S_EventStatus','varname','EventStatus','type','UInt8'},'date',735284.44087454863}, dt=-1}
      mask help:
      | TargetLink Custom Code block:
      | Allows to insert custom code into a TargetLink application.
      settings: AttributesFormatString=Dem_SetEventStatusDep  DeleteFcn=if exist('delete_tlblock','file')==2,delete_tlblock(gcbh);end  NameChangeFcn=if exist('rename_tlblock','file')==2,rename_tlblock(gcbh);end  OpenFcn=if exist('tl_open_blockdlg','file')==2,tl_open_blockdlg(gcbh);else,open_system(gcbh,'mask');end
      mask Help: eval(['tl_online_help(''Topic'',''',get_param(gcbh,'MaskType'),''')'])
      mask Display:
      | plot([-0.05, 1.05, NaN, -0.05, 1.05],[.01, .01, NaN, .99, .99])
      | ; disp('Dem_SetEventStatusDep.c');port_label('input',1,'EventId');port_label('input',2,'EventStatus');port_label('output',1,'ok');
  Pre-Failed : Constant  Value=3  mask(TL_Constant){data={'date',735284.44036082178}}
      settings: CopyFcn=if exist('tl_reset_reviewflag','file')==2,tl_reset_reviewflag(gcbh);end  DeleteFcn=if exist('delete_tlblock','file')==2,delete_tlblock(gcbh);end  NameChangeFcn=if exist('rename_tlblock','file')==2,rename_tlblock(gcbh);end  OpenFcn=if exist('tl_open_blockdlg','file')==2,tl_open_blockdlg(gcbh);else,open_system(gcbh,'parameter');end
      mask Help: eval(['if exist(''tl_online_help'',''file'') == 2, tl_online_help(''Topic'',''TL_Constant''),else, web([''jar:file:///'',matlabroot,''/help/toolbox/simulink/help.jar!/slref/' lower(get_param(gcbh,'Blocktype')) '.html''], ''-helpbrowser''),end'])
      mask Display: plot([-0.05, 1.05, NaN, -0.05, 1.05],[.01, .01, NaN, .99, .99])
  Terminator3 : Terminator
  wires:
  Pre-Failed/1 -> Dem_SetEventStatus/2
  VcEv/1 -> Dem_SetEventStatus/1
  Dem_SetEventStatus/1 -> Terminator3/1
